simulink model "BMS_Integration"  (R2020a)
settings: configuration reference "Common_config_codegen" (kept outside this file)
libraries: simulink x2
settings Model: DataDictionary=Common.sldd  Creator="wei  zhao"  LastModifiedBy="wei  zhao"
settings ConfigSetRef: SourceName=Common_config_codegen

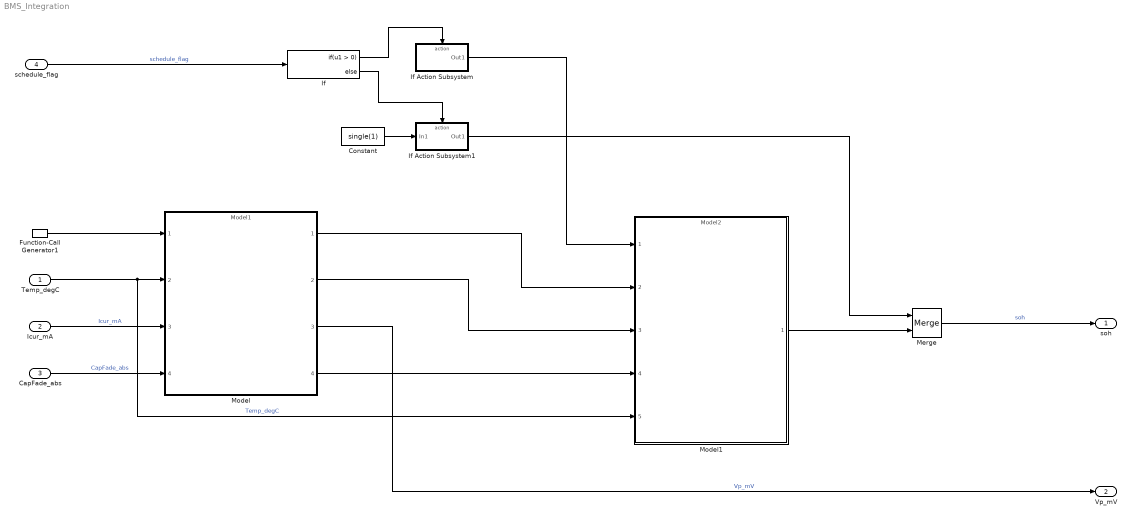
== system BMS_Integration ==
  Temp_degC : Inport
  Icur_mA : Inport  Port=2
  CapFade_abs : Inport  Port=3
  schedule_flag : Inport  Port=4
  Constant : Constant  Value=single(1)
  Function-Call Generator1 : simulink/Ports & Subsystems/Function-Call Generator  sample_time=0.01  numberOfIterations=1
  If : If
  If Action Subsystem : Subsystem  TreatAsAtomicUnit=on
  If Action Subsystem1 : Subsystem  TreatAsAtomicUnit=on
  Merge : Merge
  Model : ModelReference  ModelNameDialog=Model1.slx  SimulationMode=Normal  ScheduleRates=on  ModelReferenceVersion=1.47
  Model1 : ModelReference  ModelNameDialog=Model2.slx  SimulationMode=Normal  ScheduleRates=on  ModelReferenceVersion=1.42
  soh : Outport
  Vp_mV : Outport  Port=2
  wires:
  Function-Call Generator1/1 -> Model/1
  Temp_degC/1 -> Model1/5, Model/2  "Temp_degC"
  Icur_mA/1 -> Model/3  "Icur_mA"
  CapFade_abs/1 -> Model/4  "CapFade_abs"
  Model/1 -> Model1/2
  Model/2 -> Model1/3
  schedule_flag/1 -> If/1  "schedule_flag"
  If/2 -> If Action Subsystem1/Action
  Constant/1 -> If Action Subsystem1/1(In1)
  Merge/1 -> soh/1  "soh"
  If/1 -> If Action Subsystem/Action
  If Action Subsystem/1(Out1) -> Model1/1
  Model/3 -> Vp_mV/1  "Vp_mV"
  Model/4 -> Model1/4
  Model1/1 -> Merge/2
  If Action Subsystem1/1(Out1) -> Merge/1

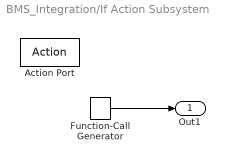
== system BMS_Integration/If Action Subsystem ==
  Action Port : ActionPort  ActionPortLabel=if(u1 > 0)
  Function-Call Generator : simulink/Ports & Subsystems/Function-Call Generator  sample_time=-1  numberOfIterations=1
  Out1 : Outport
  wires:
  Function-Call Generator/1 -> Out1/1

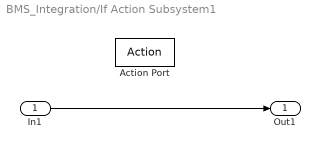
== system BMS_Integration/If Action Subsystem1 ==
  In1 : Inport
  Action Port : ActionPort  ActionPortLabel=else
  Out1 : Outport
  wires:
  In1/1 -> Out1/1
